simulink model "simulation_prev"  (R2021b)
settings: Solver=ode45  StartTime=0.0  StopTime=20.0  RelTol=1e-3
model workspace (MAT data in the model file):
  instants = 1
values from neighbouring files (symbols this model uses):
  c = modNE(x2,x2,e0,m,I,A,pc)    [ct_dynamics.m]    (also in dynamic_model_3R_spatial.m = [c1;c2;c3]; dynamic_model_simulation.m = [0.4; 0.2; 0.7]; run_experiment.m = [0.4; 0.2; 0.7])
  c0bar = norm(get_c_factorization_matrix(sol(1),sol(2),sol(3),sol(4),sol(5)))/norm(sol(3:5))    [compute_vel_obs_gain.m]    (also in dynamic_model_simulation.m = 1.96239028072; red_obs_gain_computation.m = c0; run_experiment.m = 1.96239028072)
  DHTABLE = [ pi/2      0         l(1)     q1 ... (first row only)    [compute_vel_obs_gain.m]    (also in dynamic_model_3R_spatial.m = [ pi/2      0      sym('L1') sym('q1'); dynamic_model_simulation.m = [ pi/2      0         l(1)     0; red_obs_gain_computation.m = [ pi/2      0         l(1)     0; run_experiment.m = [ pi/2      0         l(1)     0)
  eta = 1    [compute_vel_obs_gain.m]    (also in dynamic_model_simulation.m; red_obs_gain_computation.m; run_experiment.m)
  g0 = 9.81    [compute_vel_obs_gain.m]    (also in dynamic_model_3R_spatial.m; dynamic_model_simulation.m; modNE.m = 0; red_obs_gain_computation.m)
  I = zeros(3,3,N)    [compute_vel_obs_gain.m]    (also in dynamic_model_simulation.m; red_obs_gain_computation.m; run_experiment.m; run_simulation.m = zeros(3,3,3))
  K0 = c0bar*(v_max+eta)/(2*lambda_1)    [compute_vel_obs_gain.m]    (also in dynamic_model_simulation.m = 31.0539244645; red_obs_gain_computation.m = 0; run_experiment.m = 103.513081548)
  Kd = 3e1    (= 30)    [dynamic_model_simulation.m]    (also in run_experiment.m = 70; run_simulation.m = 10)
  Ko = 5e1    (= 50)    [dynamic_model_simulation.m]    (also in run_experiment.m; run_simulation.m = 0.1)
  Kp = 3e2    (= 300)    [dynamic_model_simulation.m]    (also in run_experiment.m = 70; run_simulation.m = 50)
  l = [0.5 0.5 0.4]'    [compute_eeJacobian.m]    (also in compute_vel_obs_gain.m; dynamic_model_simulation.m; eeJacobian_3R_spatial.m; red_obs_gain_computation.m)
  lambda_1 = min(min_first,min_third)/2    [compute_vel_obs_gain.m]    (also in dynamic_model_simulation.m = 0.0947894822263; red_obs_gain_computation.m = min_eig/2; run_experiment.m = 0.0473947411131)
  m = [15 10 5]'    [compute_vel_obs_gain.m]    (also in dynamic_model_simulation.m; red_obs_gain_computation.m; run_experiment.m; run_simulation.m = [m1 m2 m3]')
  pc = [0             -l(2)+dc(2) -l(3)+dc(3) ... (first row only)    [compute_vel_obs_gain.m]    (also in dynamic_model_simulation.m; red_obs_gain_computation.m; run_experiment.m)
  q0 = inverse_kinematics(p_init,l,soln_type)    [dynamic_model_simulation.m]    (also in run_experiment.m; run_simulation.m = [0,0,0]')
  r_c = 0.3    [dynamic_model_simulation.m]    (also in run_experiment.m)
  s0 = ceil(norm(dq0)/vbar)    [dynamic_model_simulation.m]
  T = simplify(T)    [DHMatrix.m]    (also in DHMatrix_sym.m; dynamic_model_3R_spatial.m = simplify(T1+T2+T3); dynamic_model_simulation.m = 2; run_experiment.m = 2)
  t0 = 2    [dynamic_model_simulation.m]    (also in run_experiment.m)
  T0 = 0.5*x2hat0'*M0*x2hat0    [dynamic_model_simulation.m]    (also in run_experiment.m)
  vbar = 2*eta+1    (= 3)    [dynamic_model_simulation.m]
  x0 = [pi/4,pi/4,1,1,1]'    [compute_vel_obs_gain.m]    (also in dynamic_model_simulation.m = [q0; dq0]; find_c0.m; run_experiment.m = [q0; dq0])
  z0 = [0 0 1]'    [dynamic_model_3R_spatial.m]    (also in dynamic_model_simulation.m = x2hat0 - K0*q0; run_experiment.m = x2hat0 - K0*q0)
undefined symbols (not defined in the file or in its folder): Levenberg, Marquardt, p_f, p_i, t_fin, t_init, time_int, trvec2tform
libraries: robotcorelib x3, SignalEditorBlockLib x1, robotmaniplib x1, matrix_library x1
(part 1 of 2)
settings Model: Creator=PcWork  LastModifiedBy=mluser
settings DataIOCC: SaveFormat=Array  SaveState=on
settings DebuggingCC: UnconnectedInputMsg=none  UnconnectedOutputMsg=none  UnconnectedLineMsg=none
settings RTWCC: DLArmComputeVersion=20.02.1

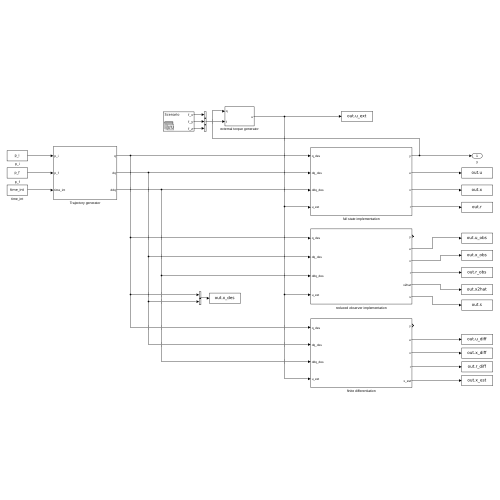
[thumbnail: Simulink's stored preview of the top-level diagram]
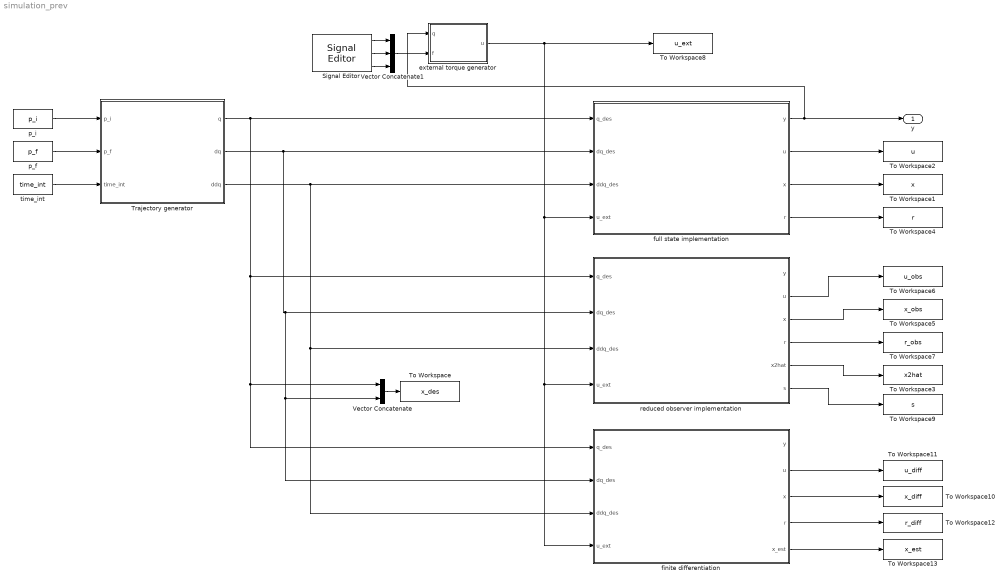
== system simulation_prev ==
  Signal Editor : SignalEditorBlockLib/Signal Editor  FileName=external_force.mat  ActiveScenario=Scenario  ActiveSignal=f_y  IsBus=off  OutputBusObjectStr=Bus: BusObject  SampleTime=0  ZeroCross=off  OutputAfterFinalValue=Setting to zero  Unit=inherit  PreserveSignalName=on
  To Workspace : ToWorkspace  VariableName=x_des  SampleTime=-1
  To Workspace1 : ToWorkspace  VariableName=x  SampleTime=-1
  To Workspace10 : ToWorkspace  VariableName=x_diff  SampleTime=-1
  To Workspace11 : ToWorkspace  VariableName=u_diff  SampleTime=-1
  To Workspace12 : ToWorkspace  VariableName=r_diff  SampleTime=-1
  To Workspace13 : ToWorkspace  VariableName=x_est  SampleTime=-1
  To Workspace2 : ToWorkspace  VariableName=u  SampleTime=-1
  To Workspace3 : ToWorkspace  VariableName=x2hat  SampleTime=-1
  To Workspace4 : ToWorkspace  VariableName=r  SampleTime=-1
  To Workspace5 : ToWorkspace  VariableName=x_obs  SampleTime=-1
  To Workspace6 : ToWorkspace  VariableName=u_obs  SampleTime=-1
  To Workspace7 : ToWorkspace  VariableName=r_obs  SampleTime=-1
  To Workspace8 : ToWorkspace  VariableName=u_ext  SampleTime=-1
  To Workspace9 : ToWorkspace  VariableName=s  SampleTime=-1
  Trajectory generator : Subsystem
  Vector Concatenate : Concatenate
  Vector Concatenate1 : Concatenate  NumInputs=3
  external torque generator : Subsystem
  finite differentiation : Subsystem
  full state implementation : Subsystem
  p_f : Constant  Value=p_f
  p_i : Constant  Value=p_i
  reduced observer implementation : Subsystem
  time_int : Constant  Value=time_int
  y : Outport
  wires:
  full state implementation/2(u) -> To Workspace2/1
  full state implementation/4(r) -> To Workspace4/1
  full state implementation/1(y) -> y/1, external torque generator/1(q)
  Vector Concatenate/1 -> To Workspace/1
  full state implementation/3(x) -> To Workspace1/1
  reduced observer implementation/2(u) -> To Workspace6/1
  reduced observer implementation/3(x) -> To Workspace5/1
  reduced observer implementation/4(r) -> To Workspace7/1
  external torque generator/1(u) -> finite differentiation/4(u_ext), reduced observer implementation/4(u_ext), full state implementation/4(u_ext), To Workspace8/1
  reduced observer implementation/5(x2hat) -> To Workspace3/1
  reduced observer implementation/6(s) -> To Workspace9/1
  finite differentiation/2(u) -> To Workspace11/1
  finite differentiation/3(x) -> To Workspace10/1
  finite differentiation/4(r) -> To Workspace12/1
  finite differentiation/5(x_est) -> To Workspace13/1
  Signal Editor/2 -> Vector Concatenate1/2
  Signal Editor/3 -> Vector Concatenate1/3
  Vector Concatenate1/1 -> external torque generator/2(f)
  Signal Editor/1 -> Vector Concatenate1/1
  p_i/1 -> Trajectory generator/1(p_i)
  p_f/1 -> Trajectory generator/2(p_f)
  time_int/1 -> Trajectory generator/3(time_int)
  Trajectory generator/1(q) -> finite differentiation/1(q_des), Vector Concatenate/1, reduced observer implementation/1(q_des), full state implementation/1(q_des)
  Trajectory generator/2(dq) -> full state implementation/2(dq_des), reduced observer implementation/2(dq_des), finite differentiation/2(dq_des), Vector Concatenate/2
  Trajectory generator/3(ddq) -> full state implementation/3(ddq_des), finite differentiation/3(ddq_des), reduced observer implementation/3(ddq_des)

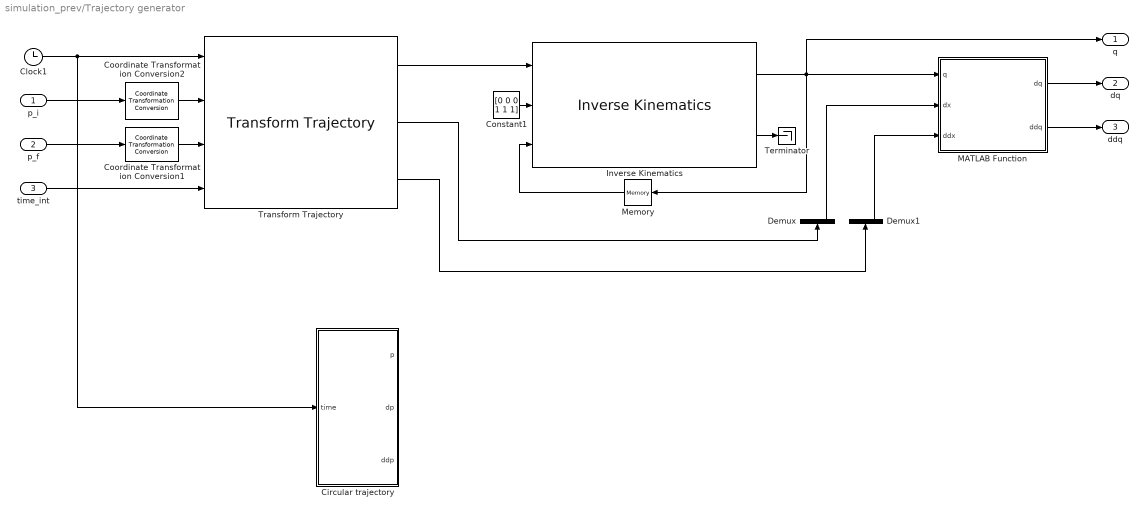
== system simulation_prev/Trajectory generator ==
  p_i : Inport
  p_f : Inport  Port=2
  time_int : Inport  Port=3
  Circular trajectory : Subsystem
  Clock1 : Clock
  Constant1 : Constant  Value=[0 0 0 1 1 1]
  Coordinate Transformation Conversion1 : robotcorelib/Coordinate Transformation Conversion  InputRepresentation=Translation Vector  InputEulerSequence=ZYX  ShowTrVecInputPort=on  OutputRepresentation=Homogeneous Transformation  OutputEulerSequence=ZYX  ShowTrVecOutputPort=on  SimulateUsing=Interpreted execution
  Coordinate Transformation Conversion2 : robotcorelib/Coordinate Transformation Conversion  InputRepresentation=Translation Vector  InputEulerSequence=ZYX  ShowTrVecInputPort=on  OutputRepresentation=Homogeneous Transformation  OutputEulerSequence=ZYX  ShowTrVecOutputPort=on  SimulateUsing=Interpreted execution
  Demux : Demux  Outputs=2
  Demux1 : Demux  Outputs=2
  Inverse Kinematics : robotmaniplib/Inverse Kinematics  RigidBodyTree=robot  EndEffector=body3  ShowInfo=on  SolverName=Levenberg-Marquardt  EnforceJointLimits=on  MaxIterations=1500  MaxTime=10  GradientTolerance=1e-3  SolutionTolerance=1e-2  StepTolerance=1e-14  ErrorChangeTolerance=1e-3  UseErrorDamping=on  DampingBias=0.0025  SimulateUsing=Interpreted execution
  MATLAB Function : MATLAB Function  TreatAsAtomicUnit=on
  Memory : Memory  InitialCondition=q0  InheritSampleTime=on
  Terminator : Terminator
  Transform Trajectory : robotcorelib/Transform Trajectory  WaypointSource=External  T0=trvec2tform(p_i)  TF=trvec2tform(p_f)  TimeInterval=time_int  CustomTimeScaling=off  ParameterSource=Internal  TSTime=2:0.1:3  TimeScaling=[ 0:0.1:1; ones( 1, 11 ); zeros( 1, 11 ) ]  SimulateUsing=Interpreted execution
  q : Outport
  dq : Outport  Port=2
  ddq : Outport  Port=3
  wires:
  time_int/1 -> Transform Trajectory/4
  Inverse Kinematics/1 -> q/1, MATLAB Function/1(q), Memory/1
  Transform Trajectory/1 -> Inverse Kinematics/1
  Demux/2 -> MATLAB Function/2(dx)
  Transform Trajectory/3 -> Demux1/1
  MATLAB Function/2(ddq) -> ddq/1
  MATLAB Function/1(dq) -> dq/1
  p_f/1 -> Coordinate Transformation Conversion1/1
  Clock1/1 -> Circular trajectory/1(time), Transform Trajectory/1
  p_i/1 -> Coordinate Transformation Conversion2/1
  Coordinate Transformation Conversion2/1 -> Transform Trajectory/2
  Coordinate Transformation Conversion1/1 -> Transform Trajectory/3
  Memory/1 -> Inverse Kinematics/3
  Transform Trajectory/2 -> Demux/1
  Demux1/2 -> MATLAB Function/3(ddx)
  Constant1/1 -> Inverse Kinematics/2
  Inverse Kinematics/2 -> Terminator/1

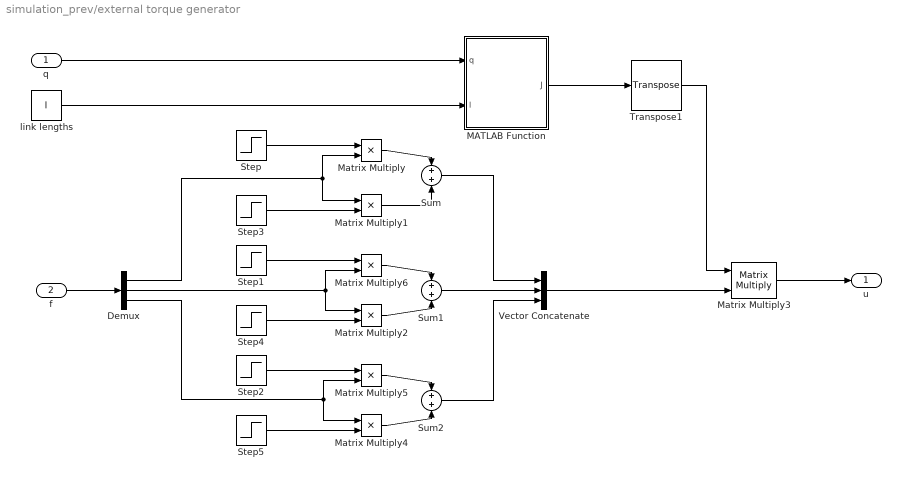
== system simulation_prev/external torque generator ==
  q : Inport
  f : Inport  Port=2
  Demux : Demux  Outputs=3
  MATLAB Function : MATLAB Function  TreatAsAtomicUnit=on
  Matrix Multiply{,1..2,4..6} (6 alike) : Product
  Matrix Multiply3 : Product  Multiplication=Matrix(*)
  Step : Step  Time=t_init  SampleTime=0
  Step1 : Step  Time=t_init  SampleTime=0
  Step2 : Step  Time=t_init  SampleTime=0
  Step3 : Step  Time=t_fin  After=-1  SampleTime=0
  Step4 : Step  Time=t_fin  After=-1  SampleTime=0
  Step5 : Step  Time=t_fin  After=-1  SampleTime=0
  Sum : Sum
  Sum1 : Sum
  Sum2 : Sum
  Transpose1 : matrix_library/Transpose
  Vector Concatenate : Concatenate  NumInputs=3
  link lengths : Constant  Value=l
  u : Outport
  wires:
  Step1/1 -> Matrix Multiply6/1
  Demux/2 -> Matrix Multiply2/1, Matrix Multiply6/2
  Demux/1 -> Matrix Multiply1/1, Matrix Multiply/2
  f/1 -> Demux/1
  MATLAB Function/1(J) -> Transpose1/1
  Transpose1/1 -> Matrix Multiply3/1
  Vector Concatenate/1 -> Matrix Multiply3/2
  Matrix Multiply3/1 -> u/1
  q/1 -> MATLAB Function/1(q)
  link lengths/1 -> MATLAB Function/2(l)
  Step3/1 -> Matrix Multiply1/2
  Step4/1 -> Matrix Multiply2/2
  Step/1 -> Matrix Multiply/1
  Matrix Multiply1/1 -> Sum/2
  Sum/1 -> Vector Concatenate/1
  Matrix Multiply/1 -> Sum/1
  Matrix Multiply6/1 -> Sum1/1
  Matrix Multiply2/1 -> Sum1/2
  Sum1/1 -> Vector Concatenate/2
  Step5/1 -> Matrix Multiply4/2
  Matrix Multiply5/1 -> Sum2/1
  Demux/3 -> Matrix Multiply5/2, Matrix Multiply4/1
  Matrix Multiply4/1 -> Sum2/2
  Step2/1 -> Matrix Multiply5/1
  Sum2/1 -> Vector Concatenate/3

== system simulation_prev/finite differentiation ==
  q_des : Inport
  dq_des : Inport  Port=2
  ddq_des : Inport  Port=3
  u_ext : Inport  Port=4
  Controller : Subsystem
  Demux1 : Demux  Outputs=2
  Derivative : Derivative
  Robot dynamics : Subsystem
  Sum : Sum
  Terminator : Terminator
  Vector Concatenate : Concatenate
  energy residual : Subsystem
  y : Outport
  u : Outport  Port=2
  x : Outport  Port=3
  r : Outport  Port=4
  x_est : Outport  Port=5
  wires:
  Demux1/1 -> Derivative/1, Vector Concatenate/1, y/1
  energy residual/1(r) -> r/1
  q_des/1 -> Controller/2(q_des)
  Controller/1(u) -> energy residual/2(u_m), Sum/1, u/1
  ddq_des/1 -> Controller/4(ddq_des)
  Demux1/2 -> Terminator/1
  dq_des/1 -> Controller/3(dq_des)
  Robot dynamics/1(x) -> x/1, Demux1/1
  Vector Concatenate/1 -> x_est/1, energy residual/1(x), Controller/1(x)
  Sum/1 -> Robot dynamics/1(u)
  u_ext/1 -> Sum/2
  Derivative/1 -> Vector Concatenate/2

== system simulation_prev/full state implementation ==
  q_des : Inport
  dq_des : Inport  Port=2
  ddq_des : Inport  Port=3
  u_ext : Inport  Port=4
  Controller : Subsystem
  Demux1 : Demux  Outputs=2
  Robot dynamics : Subsystem
  Sum : Sum
  Terminator : Terminator
  energy residual : Subsystem
  y : Outport
  u : Outport  Port=2
  x : Outport  Port=3
  r : Outport  Port=4
  wires:
  Demux1/2 -> Terminator/1
  Robot dynamics/1(x) -> energy residual/1(x), x/1, Demux1/1, Controller/1(x)
  energy residual/1(r) -> r/1
  Sum/1 -> Robot dynamics/1(u)
  q_des/1 -> Controller/2(q_des)
  Controller/1(u) -> u/1, Sum/1, energy residual/2(u_m)
  dq_des/1 -> Controller/3(dq_des)
  ddq_des/1 -> Controller/4(ddq_des)
  Demux1/1 -> y/1
  u_ext/1 -> Sum/2

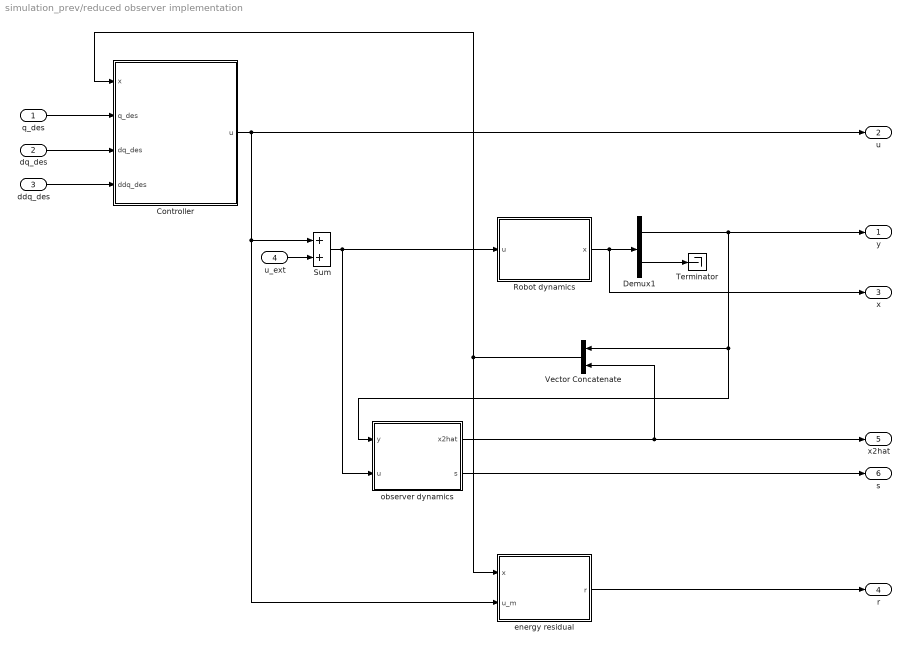
== system simulation_prev/reduced observer implementation ==
  q_des : Inport
  dq_des : Inport  Port=2
  ddq_des : Inport  Port=3
  u_ext : Inport  Port=4
  Controller : Subsystem
  Demux1 : Demux  Outputs=2
  Robot dynamics : Subsystem
  Sum : Sum
  Terminator : Terminator
  Vector Concatenate : Concatenate
  energy residual : Subsystem
  observer dynamics : Subsystem
  y : Outport
  u : Outport  Port=2
  x : Outport  Port=3
  r : Outport  Port=4
  x2hat : Outport  Port=5
  s : Outport  Port=6
  wires:
  Demux1/1 -> Vector Concatenate/1, observer dynamics/1(y), y/1
  observer dynamics/1(x2hat) -> x2hat/1, Vector Concatenate/2
  energy residual/1(r) -> r/1
  q_des/1 -> Controller/2(q_des)
  Controller/1(u) -> energy residual/2(u_m), Sum/1, u/1
  ddq_des/1 -> Controller/4(ddq_des)
  Demux1/2 -> Terminator/1
  dq_des/1 -> Controller/3(dq_des)
  Robot dynamics/1(x) -> x/1, Demux1/1
  Vector Concatenate/1 -> energy residual/1(x), Controller/1(x)
  Sum/1 -> Robot dynamics/1(u), observer dynamics/2(u)
  u_ext/1 -> Sum/2
  observer dynamics/2(s) -> s/1

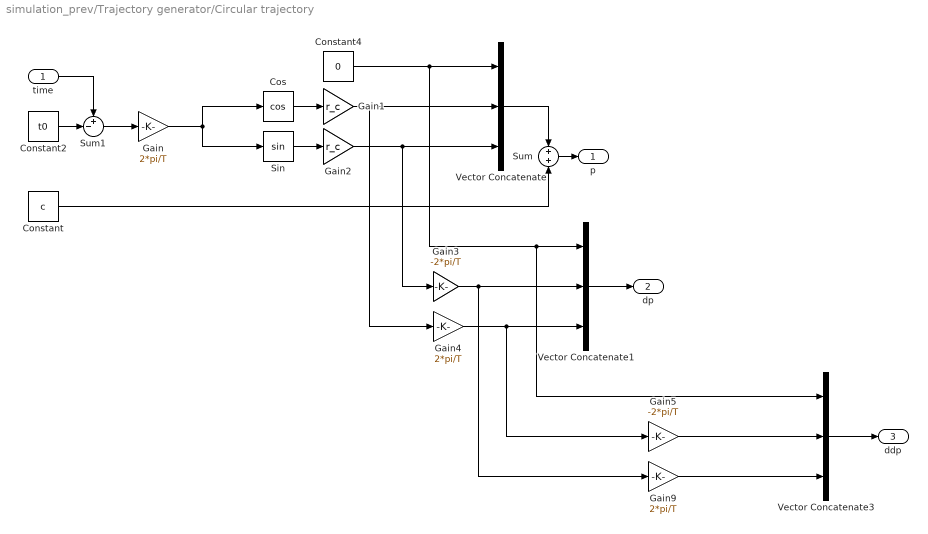
== system simulation_prev/Trajectory generator/Circular trajectory ==
  time : Inport
  Constant : Constant  Value=c
  Constant2 : Constant  Value=t0
  Constant4 : Constant  Value=0
  Cos : Trigonometry  Operator=cos
  Gain : Gain  Gain=2*pi/T
  Gain1 : Gain  Gain=r_c
  Gain2 : Gain  Gain=r_c
  Gain3 : Gain  Gain=-2*pi/T
  Gain4 : Gain  Gain=2*pi/T
  Gain5 : Gain  Gain=-2*pi/T
  Gain9 : Gain  Gain=2*pi/T
  Sin : Trigonometry
  Sum : Sum
  Sum1 : Sum  Inputs=+-|
  Vector Concatenate : Concatenate  NumInputs=3
  Vector Concatenate1 : Concatenate  NumInputs=3
  Vector Concatenate3 : Concatenate  NumInputs=3
  p : Outport
  dp : Outport  Port=2
  ddp : Outport  Port=3
  wires:
  Constant2/1 -> Sum1/2
  Sum/1 -> p/1
  Sum1/1 -> Gain/1
  Constant4/1 -> Vector Concatenate3/1, Vector Concatenate1/1, Vector Concatenate/1
  Gain2/1 -> Vector Concatenate/3, Gain3/1
  Constant/1 -> Sum/2
  time/1 -> Sum1/1
  Cos/1 -> Gain1/1
  Gain/1 -> Sin/1, Cos/1
  Sin/1 -> Gain2/1
  Vector Concatenate/1 -> Sum/1
  Gain1/1 -> Vector Concatenate/2, Gain4/1
  Gain3/1 -> Gain9/1, Vector Concatenate1/2
  Gain4/1 -> Gain5/1, Vector Concatenate1/3
  Gain9/1 -> Vector Concatenate3/3
  Gain5/1 -> Vector Concatenate3/2
  Vector Concatenate3/1 -> ddp/1
  Vector Concatenate1/1 -> dp/1

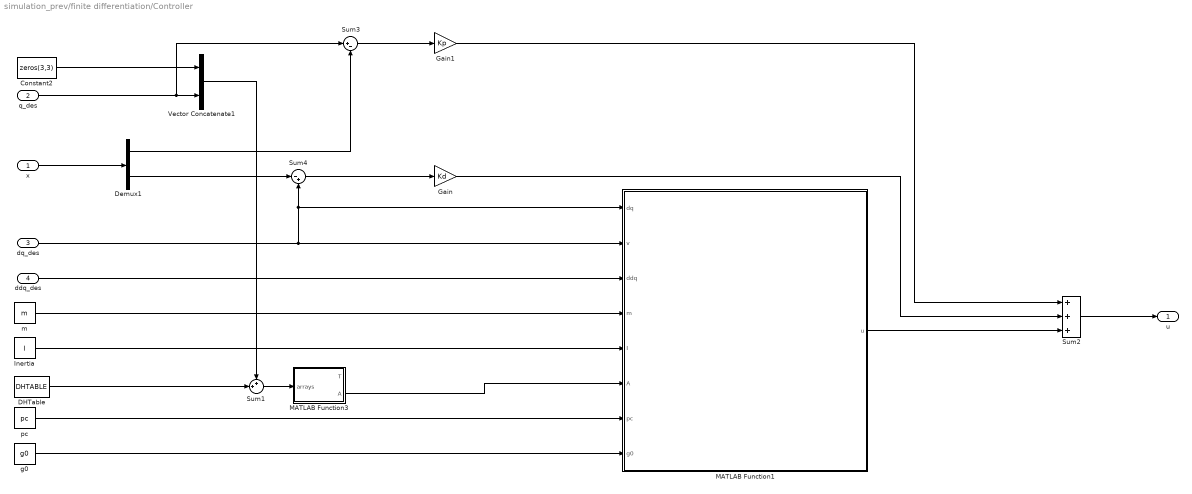
== system simulation_prev/finite differentiation/Controller ==
  x : Inport
  q_des : Inport  Port=2
  dq_des : Inport  Port=3
  ddq_des : Inport  Port=4
  Constant2 : Constant  Value=zeros(3,3)
  DHTable : Constant  Value=DHTABLE
  Demux1 : Demux  Outputs=2
  Gain : Gain  Gain=Kd
  Gain1 : Gain  Gain=Kp
  Inertia : Constant  Value=I
  MATLAB Function1 : MATLAB Function  TreatAsAtomicUnit=on
  MATLAB Function3 : MATLAB Function  TreatAsAtomicUnit=on
  Sum1 : Sum  Inputs=++|
  Sum2 : Sum  Inputs=+++
  Sum3 : Sum  Inputs=|+-
  Sum4 : Sum  Inputs=|-+
  Vector Concatenate1 : Concatenate  Mode=Multidimensional array  ConcatenateDimension=2
  g0 : Constant  Value=g0
  m : Constant  Value=m
  pc : Constant  Value=pc
  u : Outport
  wires:
  MATLAB Function3/2(A) -> MATLAB Function1/6(A)
  dq_des/1 -> MATLAB Function1/1(dq), Sum4/2, MATLAB Function1/2(v)
  ddq_des/1 -> MATLAB Function1/3(ddq)
  Sum1/1 -> MATLAB Function3/1(arrays)
  Constant2/1 -> Vector Concatenate1/1
  Sum4/1 -> Gain/1
  Vector Concatenate1/1 -> Sum1/1
  m/1 -> MATLAB Function1/4(m)
  g0/1 -> MATLAB Function1/8(g0)
  Sum3/1 -> Gain1/1
  q_des/1 -> Vector Concatenate1/2, Sum3/1
  DHTable/1 -> Sum1/2
  Inertia/1 -> MATLAB Function1/5(I)
  pc/1 -> MATLAB Function1/7(pc)
  Sum2/1 -> u/1
  MATLAB Function1/1(u) -> Sum2/3
  Gain/1 -> Sum2/2
  Gain1/1 -> Sum2/1
  x/1 -> Demux1/1
  Demux1/2 -> Sum4/1
  Demux1/1 -> Sum3/2

== system simulation_prev/finite differentiation/Robot dynamics ==
  u : Inport
  Constant : Constant  Value=zeros(3,3)
  DHTable : Constant  Value=DHTABLE
  Demux1 : Demux  Outputs=2
  Inertia : Constant  Value=I
  Integrator : Integrator  InitialConditionSource=external  InitialCondition=[0 pi/4 pi/4 0 0 0]'
  MATLAB Function : MATLAB Function  TreatAsAtomicUnit=on
  MATLAB Function2 : MATLAB Function  TreatAsAtomicUnit=on
  Sum : Sum
  Vector Concatenate : Concatenate  Mode=Multidimensional array  ConcatenateDimension=2
  g0 : Constant  Value=g0
  m : Constant  Value=m
  pc : Constant  Value=pc
  x0 : Constant  Value=x0
  x : Outport
  wires:
  Vector Concatenate/1 -> Sum/1
  Constant/1 -> Vector Concatenate/1
  Integrator/1 -> Demux1/1, MATLAB Function/1(x), x/1
  MATLAB Function/1(dx) -> Integrator/1
  x0/1 -> Integrator/2
  u/1 -> MATLAB Function/2(u)
  Sum/1 -> MATLAB Function2/1(arrays)
  MATLAB Function2/2(A) -> MATLAB Function/5(A)
  DHTable/1 -> Sum/2
  pc/1 -> MATLAB Function/6(pc)
  m/1 -> MATLAB Function/3(m)
  Inertia/1 -> MATLAB Function/4(I)
  g0/1 -> MATLAB Function/7(g0)
  Demux1/1 -> Vector Concatenate/2

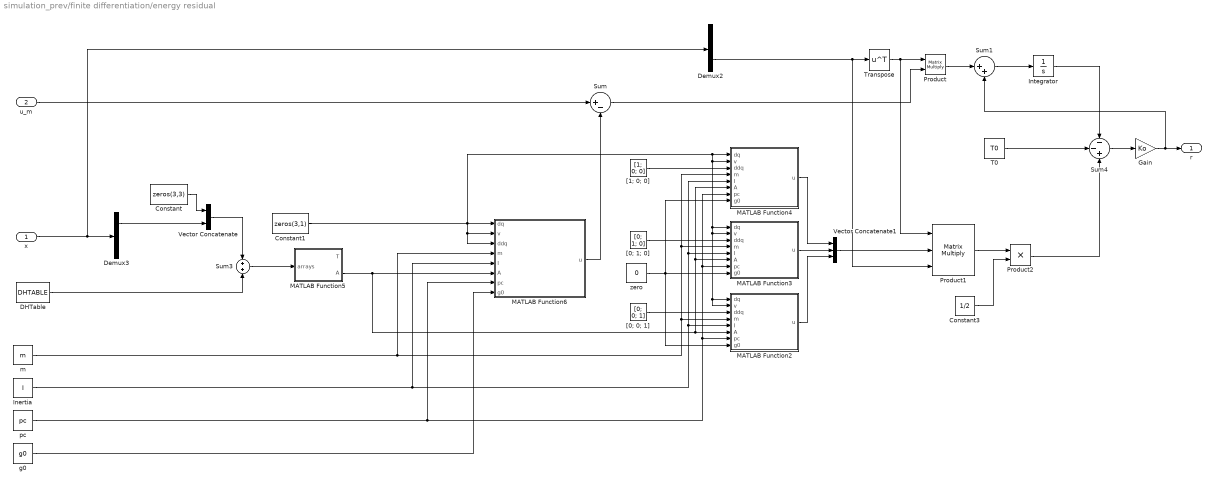
== system simulation_prev/finite differentiation/energy residual ==
  x : Inport
  u_m : Inport  Port=2
  Constant : Constant  Value=zeros(3,3)
  Constant1 : Constant  Value=zeros(3,1)
  Constant3 : Constant  Value=1/2
  DHTable : Constant  Value=DHTABLE
  Demux2 : Demux  Outputs=2
  Demux3 : Demux  Outputs=2
  Gain : Gain  Gain=Ko
  Inertia : Constant  Value=I
  Integrator : Integrator
  MATLAB Function2 : MATLAB Function  TreatAsAtomicUnit=on
  MATLAB Function3 : MATLAB Function  TreatAsAtomicUnit=on
  MATLAB Function4 : MATLAB Function  TreatAsAtomicUnit=on
  MATLAB Function5 : MATLAB Function  TreatAsAtomicUnit=on
  MATLAB Function6 : MATLAB Function  TreatAsAtomicUnit=on
  Product : Product  Multiplication=Matrix(*)
  Product1 : Product  Inputs=3  Multiplication=Matrix(*)
  Product2 : Product
  Sum : Sum  Inputs=|+-
  Sum1 : Sum  Inputs=|++
  Sum3 : Sum
  Sum4 : Sum  Inputs=--+
  T0 : Constant  Value=T0
  Transpose : Math  Operator=transpose  SaturateOnIntegerOverflow=on
  Vector Concatenate : Concatenate  Mode=Multidimensional array  ConcatenateDimension=2
  Vector Concatenate1 : Concatenate  NumInputs=3  Mode=Multidimensional array  ConcatenateDimension=2
  "[0; 0; 1]" : Constant  Value=[0; 0; 1]
  "[0; 1; 0]" : Constant  Value=[0; 1; 0]
  "[1; 0; 0]" : Constant  Value=[1; 0; 0]
  g0 : Constant  Value=g0
  m : Constant  Value=m
  pc : Constant  Value=pc
  zero : Constant  Value=0
  r : Outport
  wires:
  MATLAB Function2/1(u) -> Vector Concatenate1/3
  zero/1 -> MATLAB Function4/8(g0), MATLAB Function2/8(g0), MATLAB Function3/8(g0)
  MATLAB Function5/2(A) -> MATLAB Function6/6(A), MATLAB Function4/6(A), MATLAB Function3/6(A), MATLAB Function2/6(A)
  Sum/1 -> Product/2
  Sum1/1 -> Integrator/1
  T0/1 -> Sum4/2
  Vector Concatenate/1 -> Sum3/1
  Inertia/1 -> MATLAB Function6/5(I), MATLAB Function4/5(I), MATLAB Function3/5(I), MATLAB Function2/5(I)
  Sum4/1 -> Gain/1
  Constant/1 -> Vector Concatenate/1
  Gain/1 -> Sum1/2, r/1
  Sum3/1 -> MATLAB Function5/1(arrays)
  Constant1/1 -> MATLAB Function6/1(dq), MATLAB Function2/2(v), MATLAB Function2/1(dq), MATLAB Function3/2(v), MATLAB Function3/1(dq), MATLAB Function4/2(v), MATLAB Function4/1(dq), MATLAB Function6/2(v), MATLAB Function6/3(ddq)
  Demux3/1 -> Vector Concatenate/2
  "[1; 0; 0]"/1 -> MATLAB Function4/3(ddq)
  MATLAB Function6/1(u) -> Sum/2
  x/1 -> Demux2/1, Demux3/1
  "[0; 1; 0]"/1 -> MATLAB Function3/3(ddq)
  u_m/1 -> Sum/1
  m/1 -> MATLAB Function2/4(m), MATLAB Function3/4(m), MATLAB Function4/4(m), MATLAB Function6/4(m)
  "[0; 0; 1]"/1 -> MATLAB Function2/3(ddq)
  Constant3/1 -> Product2/2
  MATLAB Function4/1(u) -> Vector Concatenate1/1
  DHTable/1 -> Sum3/2
  MATLAB Function3/1(u) -> Vector Concatenate1/2
  Product1/1 -> Product2/1
  Vector Concatenate1/1 -> Product1/2
  Product2/1 -> Sum4/3
  g0/1 -> MATLAB Function6/8(g0)
  Demux2/2 -> Product1/3, Transpose/1
  Transpose/1 -> Product1/1, Product/1
  pc/1 -> MATLAB Function6/7(pc), MATLAB Function4/7(pc), MATLAB Function3/7(pc), MATLAB Function2/7(pc)
  Product/1 -> Sum1/1
  Integrator/1 -> Sum4/1

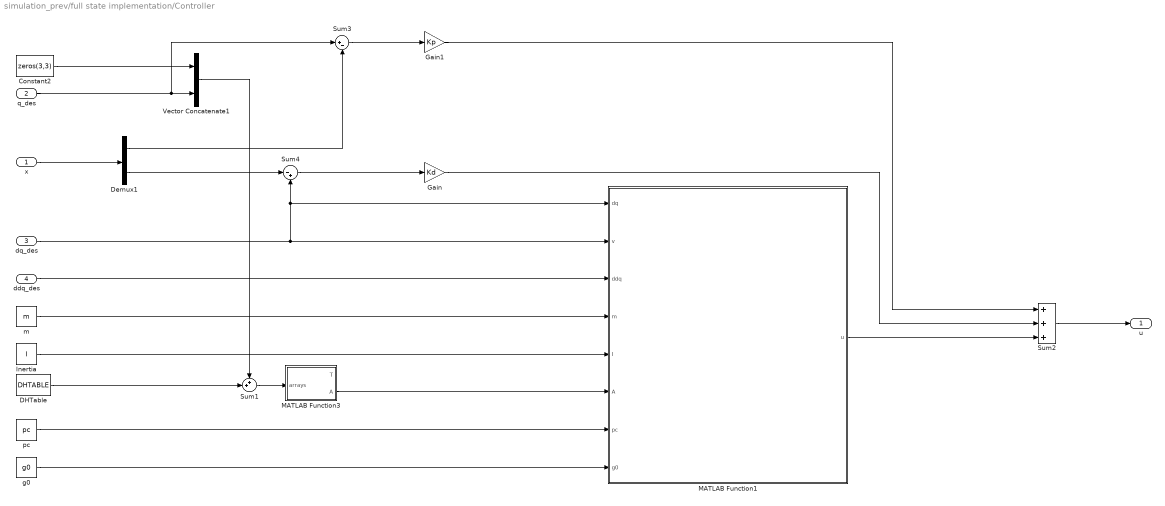
== system simulation_prev/full state implementation/Controller ==
  x : Inport
  q_des : Inport  Port=2
  dq_des : Inport  Port=3
  ddq_des : Inport  Port=4
  Constant2 : Constant  Value=zeros(3,3)
  DHTable : Constant  Value=DHTABLE
  Demux1 : Demux  Outputs=2
  Gain : Gain  Gain=Kd
  Gain1 : Gain  Gain=Kp
  Inertia : Constant  Value=I
  MATLAB Function1 : MATLAB Function  TreatAsAtomicUnit=on
  MATLAB Function3 : MATLAB Function  TreatAsAtomicUnit=on
  Sum1 : Sum  Inputs=++|
  Sum2 : Sum  Inputs=+++
  Sum3 : Sum  Inputs=|+-
  Sum4 : Sum  Inputs=|-+
  Vector Concatenate1 : Concatenate  Mode=Multidimensional array  ConcatenateDimension=2
  g0 : Constant  Value=g0
  m : Constant  Value=m
  pc : Constant  Value=pc
  u : Outport
  wires:
  MATLAB Function3/2(A) -> MATLAB Function1/6(A)
  dq_des/1 -> MATLAB Function1/1(dq), Sum4/2, MATLAB Function1/2(v)
  ddq_des/1 -> MATLAB Function1/3(ddq)
  Sum1/1 -> MATLAB Function3/1(arrays)
  Constant2/1 -> Vector Concatenate1/1
  Sum4/1 -> Gain/1
  Vector Concatenate1/1 -> Sum1/1
  m/1 -> MATLAB Function1/4(m)
  g0/1 -> MATLAB Function1/8(g0)
  Sum3/1 -> Gain1/1
  q_des/1 -> Vector Concatenate1/2, Sum3/1
  DHTable/1 -> Sum1/2
  Inertia/1 -> MATLAB Function1/5(I)
  pc/1 -> MATLAB Function1/7(pc)
  Sum2/1 -> u/1
  MATLAB Function1/1(u) -> Sum2/3
  Gain/1 -> Sum2/2
  Gain1/1 -> Sum2/1
  x/1 -> Demux1/1
  Demux1/2 -> Sum4/1
  Demux1/1 -> Sum3/2

== system simulation_prev/full state implementation/Robot dynamics ==
  u : Inport
  Constant : Constant  Value=zeros(3,3)
  DHTable : Constant  Value=DHTABLE
  Demux1 : Demux  Outputs=2
  Inertia : Constant  Value=I
  Integrator : Integrator  InitialConditionSource=external  InitialCondition=[0 pi/4 pi/4 0 0 0]'
  MATLAB Function : MATLAB Function  TreatAsAtomicUnit=on
  MATLAB Function2 : MATLAB Function  TreatAsAtomicUnit=on
  Sum : Sum
  Vector Concatenate : Concatenate  Mode=Multidimensional array  ConcatenateDimension=2
  g0 : Constant  Value=g0
  m : Constant  Value=m
  pc : Constant  Value=pc
  x0 : Constant  Value=x0
  x : Outport
  wires:
  Vector Concatenate/1 -> Sum/1
  Constant/1 -> Vector Concatenate/1
  Integrator/1 -> x/1, Demux1/1, MATLAB Function/1(x)
  MATLAB Function/1(dx) -> Integrator/1
  x0/1 -> Integrator/2
  u/1 -> MATLAB Function/2(u)
  Sum/1 -> MATLAB Function2/1(arrays)
  MATLAB Function2/2(A) -> MATLAB Function/5(A)
  DHTable/1 -> Sum/2
  pc/1 -> MATLAB Function/6(pc)
  m/1 -> MATLAB Function/3(m)
  Inertia/1 -> MATLAB Function/4(I)
  g0/1 -> MATLAB Function/7(g0)
  Demux1/1 -> Vector Concatenate/2

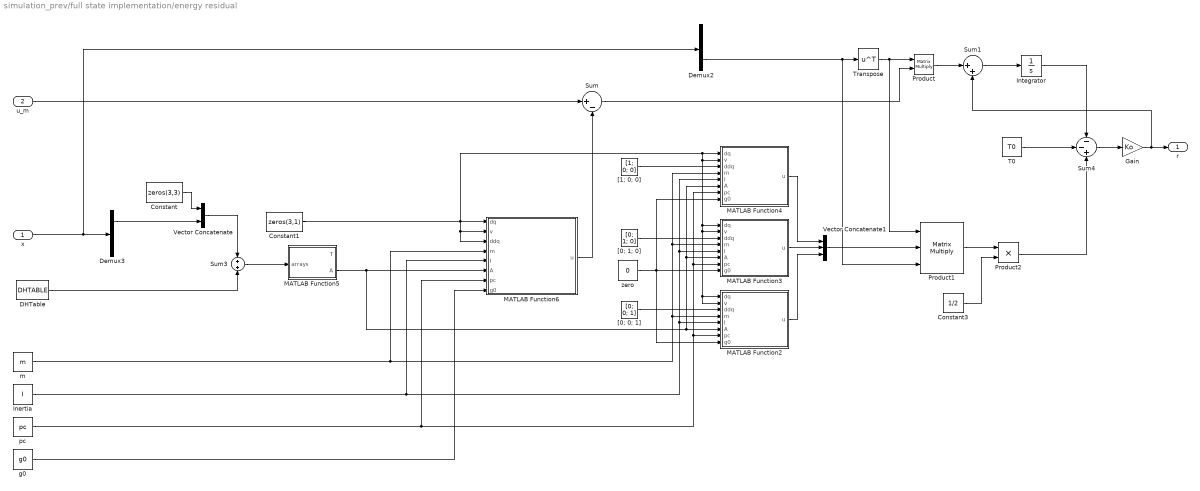
== system simulation_prev/full state implementation/energy residual ==
  x : Inport
  u_m : Inport  Port=2
  Constant : Constant  Value=zeros(3,3)
  Constant1 : Constant  Value=zeros(3,1)
  Constant3 : Constant  Value=1/2
  DHTable : Constant  Value=DHTABLE
  Demux2 : Demux  Outputs=2
  Demux3 : Demux  Outputs=2
  Gain : Gain  Gain=Ko
  Inertia : Constant  Value=I
  Integrator : Integrator
  MATLAB Function2 : MATLAB Function  TreatAsAtomicUnit=on
  MATLAB Function3 : MATLAB Function  TreatAsAtomicUnit=on
  MATLAB Function4 : MATLAB Function  TreatAsAtomicUnit=on
  MATLAB Function5 : MATLAB Function  TreatAsAtomicUnit=on
  MATLAB Function6 : MATLAB Function  TreatAsAtomicUnit=on
  Product : Product  Multiplication=Matrix(*)
  Product1 : Product  Inputs=3  Multiplication=Matrix(*)
  Product2 : Product
  Sum : Sum  Inputs=|+-
  Sum1 : Sum  Inputs=|++
  Sum3 : Sum
  Sum4 : Sum  Inputs=--+
  T0 : Constant  Value=T0
  Transpose : Math  Operator=transpose  SaturateOnIntegerOverflow=on
  Vector Concatenate : Concatenate  Mode=Multidimensional array  ConcatenateDimension=2
  Vector Concatenate1 : Concatenate  NumInputs=3  Mode=Multidimensional array  ConcatenateDimension=2
  "[0; 0; 1]" : Constant  Value=[0; 0; 1]
  "[0; 1; 0]" : Constant  Value=[0; 1; 0]
  "[1; 0; 0]" : Constant  Value=[1; 0; 0]
  g0 : Constant  Value=g0
  m : Constant  Value=m
  pc : Constant  Value=pc
  zero : Constant  Value=0
  r : Outport
  wires:
  MATLAB Function2/1(u) -> Vector Concatenate1/3
  zero/1 -> MATLAB Function4/8(g0), MATLAB Function2/8(g0), MATLAB Function3/8(g0)
  MATLAB Function5/2(A) -> MATLAB Function6/6(A), MATLAB Function4/6(A), MATLAB Function3/6(A), MATLAB Function2/6(A)
  Sum/1 -> Product/2
  Sum1/1 -> Integrator/1
  T0/1 -> Sum4/2
  Vector Concatenate/1 -> Sum3/1
  Inertia/1 -> MATLAB Function6/5(I), MATLAB Function4/5(I), MATLAB Function3/5(I), MATLAB Function2/5(I)
  Sum4/1 -> Gain/1
  Constant/1 -> Vector Concatenate/1
  Gain/1 -> Sum1/2, r/1
  Sum3/1 -> MATLAB Function5/1(arrays)
  Constant1/1 -> MATLAB Function6/1(dq), MATLAB Function2/2(v), MATLAB Function2/1(dq), MATLAB Function3/2(v), MATLAB Function3/1(dq), MATLAB Function4/2(v), MATLAB Function4/1(dq), MATLAB Function6/2(v), MATLAB Function6/3(ddq)
  Demux3/1 -> Vector Concatenate/2
  "[1; 0; 0]"/1 -> MATLAB Function4/3(ddq)
  MATLAB Function6/1(u) -> Sum/2
  x/1 -> Demux2/1, Demux3/1
  "[0; 1; 0]"/1 -> MATLAB Function3/3(ddq)
  u_m/1 -> Sum/1
  m/1 -> MATLAB Function6/4(m), MATLAB Function2/4(m), MATLAB Function3/4(m), MATLAB Function4/4(m)
  "[0; 0; 1]"/1 -> MATLAB Function2/3(ddq)
  Constant3/1 -> Product2/2
  MATLAB Function4/1(u) -> Vector Concatenate1/1
  DHTable/1 -> Sum3/2
  MATLAB Function3/1(u) -> Vector Concatenate1/2
  Product1/1 -> Product2/1
  Vector Concatenate1/1 -> Product1/2
  Product2/1 -> Sum4/3
  g0/1 -> MATLAB Function6/8(g0)
  Demux2/2 -> Product1/3, Transpose/1
  Transpose/1 -> Product1/1, Product/1
  pc/1 -> MATLAB Function6/7(pc), MATLAB Function4/7(pc), MATLAB Function3/7(pc), MATLAB Function2/7(pc)
  Product/1 -> Sum1/1
  Integrator/1 -> Sum4/1

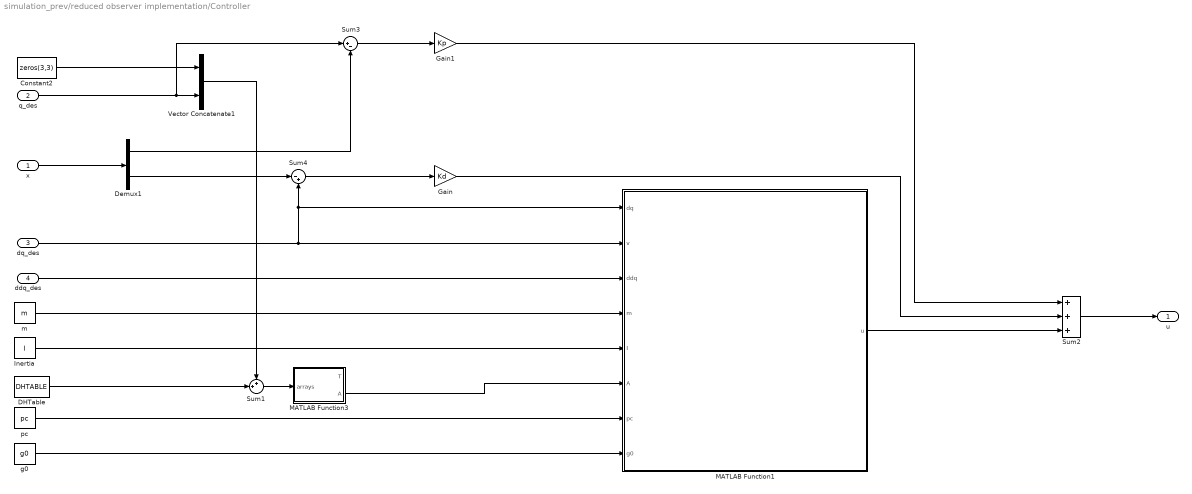
== system simulation_prev/reduced observer implementation/Controller ==
  x : Inport
  q_des : Inport  Port=2
  dq_des : Inport  Port=3
  ddq_des : Inport  Port=4
  Constant2 : Constant  Value=zeros(3,3)
  DHTable : Constant  Value=DHTABLE
  Demux1 : Demux  Outputs=2
  Gain : Gain  Gain=Kd
  Gain1 : Gain  Gain=Kp
  Inertia : Constant  Value=I
  MATLAB Function1 : MATLAB Function  TreatAsAtomicUnit=on
  MATLAB Function3 : MATLAB Function  TreatAsAtomicUnit=on
  Sum1 : Sum  Inputs=++|
  Sum2 : Sum  Inputs=+++
  Sum3 : Sum  Inputs=|+-
  Sum4 : Sum  Inputs=|-+
  Vector Concatenate1 : Concatenate  Mode=Multidimensional array  ConcatenateDimension=2
  g0 : Constant  Value=g0
  m : Constant  Value=m
  pc : Constant  Value=pc
  u : Outport
  wires:
  MATLAB Function3/2(A) -> MATLAB Function1/6(A)
  dq_des/1 -> MATLAB Function1/1(dq), Sum4/2, MATLAB Function1/2(v)
  ddq_des/1 -> MATLAB Function1/3(ddq)
  Sum1/1 -> MATLAB Function3/1(arrays)
  Constant2/1 -> Vector Concatenate1/1
  Sum4/1 -> Gain/1
  Vector Concatenate1/1 -> Sum1/1
  m/1 -> MATLAB Function1/4(m)
  g0/1 -> MATLAB Function1/8(g0)
  Sum3/1 -> Gain1/1
  q_des/1 -> Vector Concatenate1/2, Sum3/1
  DHTable/1 -> Sum1/2
  Inertia/1 -> MATLAB Function1/5(I)
  pc/1 -> MATLAB Function1/7(pc)
  Sum2/1 -> u/1
  MATLAB Function1/1(u) -> Sum2/3
  Gain/1 -> Sum2/2
  Gain1/1 -> Sum2/1
  x/1 -> Demux1/1
  Demux1/2 -> Sum4/1
  Demux1/1 -> Sum3/2

== system simulation_prev/reduced observer implementation/Robot dynamics ==
  u : Inport
  Constant : Constant  Value=zeros(3,3)
  DHTable : Constant  Value=DHTABLE
  Demux1 : Demux  Outputs=2
  Inertia : Constant  Value=I
  Integrator : Integrator  InitialConditionSource=external  InitialCondition=[0 pi/4 pi/4 0 0 0]'
  MATLAB Function : MATLAB Function  TreatAsAtomicUnit=on
  MATLAB Function2 : MATLAB Function  TreatAsAtomicUnit=on
  Sum : Sum
  Vector Concatenate : Concatenate  Mode=Multidimensional array  ConcatenateDimension=2
  g0 : Constant  Value=g0
  m : Constant  Value=m
  pc : Constant  Value=pc
  x0 : Constant  Value=x0
  x : Outport
  wires:
  Vector Concatenate/1 -> Sum/1
  Constant/1 -> Vector Concatenate/1
  Integrator/1 -> Demux1/1, MATLAB Function/1(x), x/1
  MATLAB Function/1(dx) -> Integrator/1
  x0/1 -> Integrator/2
  u/1 -> MATLAB Function/2(u)
  Sum/1 -> MATLAB Function2/1(arrays)
  MATLAB Function2/2(A) -> MATLAB Function/5(A)
  DHTable/1 -> Sum/2
  pc/1 -> MATLAB Function/6(pc)
  m/1 -> MATLAB Function/3(m)
  Inertia/1 -> MATLAB Function/4(I)
  g0/1 -> MATLAB Function/7(g0)
  Demux1/1 -> Vector Concatenate/2

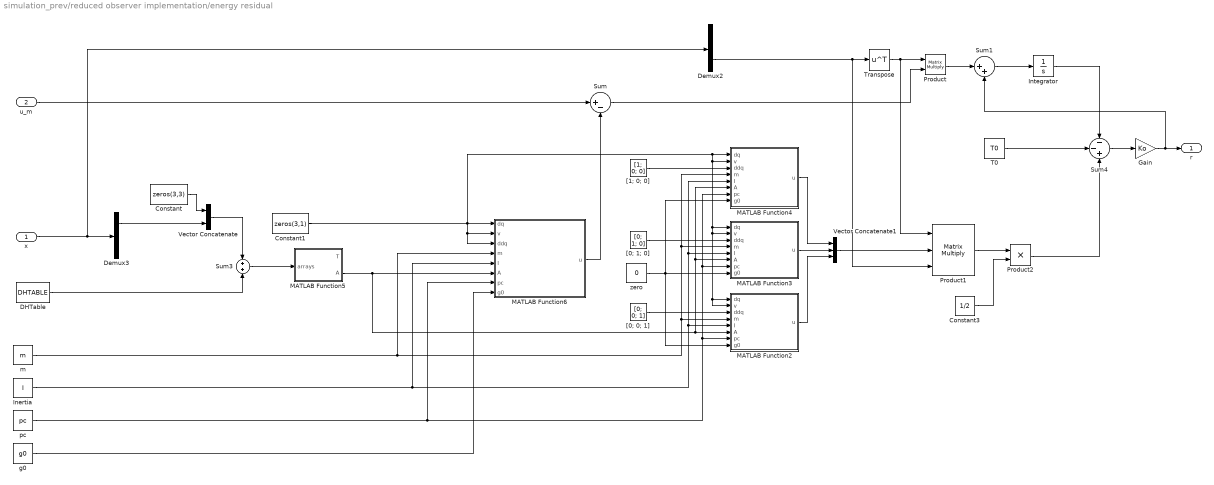
== system simulation_prev/reduced observer implementation/energy residual ==
  x : Inport
  u_m : Inport  Port=2
  Constant : Constant  Value=zeros(3,3)
  Constant1 : Constant  Value=zeros(3,1)
  Constant3 : Constant  Value=1/2
  DHTable : Constant  Value=DHTABLE
  Demux2 : Demux  Outputs=2
  Demux3 : Demux  Outputs=2
  Gain : Gain  Gain=Ko
  Inertia : Constant  Value=I
  Integrator : Integrator
  MATLAB Function2 : MATLAB Function  TreatAsAtomicUnit=on
  MATLAB Function3 : MATLAB Function  TreatAsAtomicUnit=on
  MATLAB Function4 : MATLAB Function  TreatAsAtomicUnit=on
  MATLAB Function5 : MATLAB Function  TreatAsAtomicUnit=on
  MATLAB Function6 : MATLAB Function  TreatAsAtomicUnit=on
  Product : Product  Multiplication=Matrix(*)
  Product1 : Product  Inputs=3  Multiplication=Matrix(*)
  Product2 : Product
  Sum : Sum  Inputs=|+-
  Sum1 : Sum  Inputs=|++
  Sum3 : Sum
  Sum4 : Sum  Inputs=--+
  T0 : Constant  Value=T0
  Transpose : Math  Operator=transpose  SaturateOnIntegerOverflow=on
  Vector Concatenate : Concatenate  Mode=Multidimensional array  ConcatenateDimension=2
  Vector Concatenate1 : Concatenate  NumInputs=3  Mode=Multidimensional array  ConcatenateDimension=2
  "[0; 0; 1]" : Constant  Value=[0; 0; 1]
  "[0; 1; 0]" : Constant  Value=[0; 1; 0]
  "[1; 0; 0]" : Constant  Value=[1; 0; 0]
  g0 : Constant  Value=g0
  m : Constant  Value=m
  pc : Constant  Value=pc
  zero : Constant  Value=0
  r : Outport
  wires:
  MATLAB Function2/1(u) -> Vector Concatenate1/3
  zero/1 -> MATLAB Function4/8(g0), MATLAB Function2/8(g0), MATLAB Function3/8(g0)
  MATLAB Function5/2(A) -> MATLAB Function6/6(A), MATLAB Function4/6(A), MATLAB Function3/6(A), MATLAB Function2/6(A)
  Sum/1 -> Product/2
  Sum1/1 -> Integrator/1
  T0/1 -> Sum4/2
  Vector Concatenate/1 -> Sum3/1
  Inertia/1 -> MATLAB Function6/5(I), MATLAB Function4/5(I), MATLAB Function3/5(I), MATLAB Function2/5(I)
  Sum4/1 -> Gain/1
  Constant/1 -> Vector Concatenate/1
  Gain/1 -> Sum1/2, r/1
  Sum3/1 -> MATLAB Function5/1(arrays)
  Constant1/1 -> MATLAB Function6/1(dq), MATLAB Function2/2(v), MATLAB Function2/1(dq), MATLAB Function3/2(v), MATLAB Function3/1(dq), MATLAB Function4/2(v), MATLAB Function4/1(dq), MATLAB Function6/2(v), MATLAB Function6/3(ddq)
  Demux3/1 -> Vector Concatenate/2
  "[1; 0; 0]"/1 -> MATLAB Function4/3(ddq)
  MATLAB Function6/1(u) -> Sum/2
  x/1 -> Demux2/1, Demux3/1
  "[0; 1; 0]"/1 -> MATLAB Function3/3(ddq)
  u_m/1 -> Sum/1
  m/1 -> MATLAB Function2/4(m), MATLAB Function3/4(m), MATLAB Function4/4(m), MATLAB Function6/4(m)
  "[0; 0; 1]"/1 -> MATLAB Function2/3(ddq)
  Constant3/1 -> Product2/2
  MATLAB Function4/1(u) -> Vector Concatenate1/1
  DHTable/1 -> Sum3/2
  MATLAB Function3/1(u) -> Vector Concatenate1/2
  Product1/1 -> Product2/1
  Vector Concatenate1/1 -> Product1/2
  Product2/1 -> Sum4/3
  g0/1 -> MATLAB Function6/8(g0)
  Demux2/2 -> Product1/3, Transpose/1
  Transpose/1 -> Product1/1, Product/1
  pc/1 -> MATLAB Function6/7(pc), MATLAB Function4/7(pc), MATLAB Function3/7(pc), MATLAB Function2/7(pc)
  Product/1 -> Sum1/1
  Integrator/1 -> Sum4/1

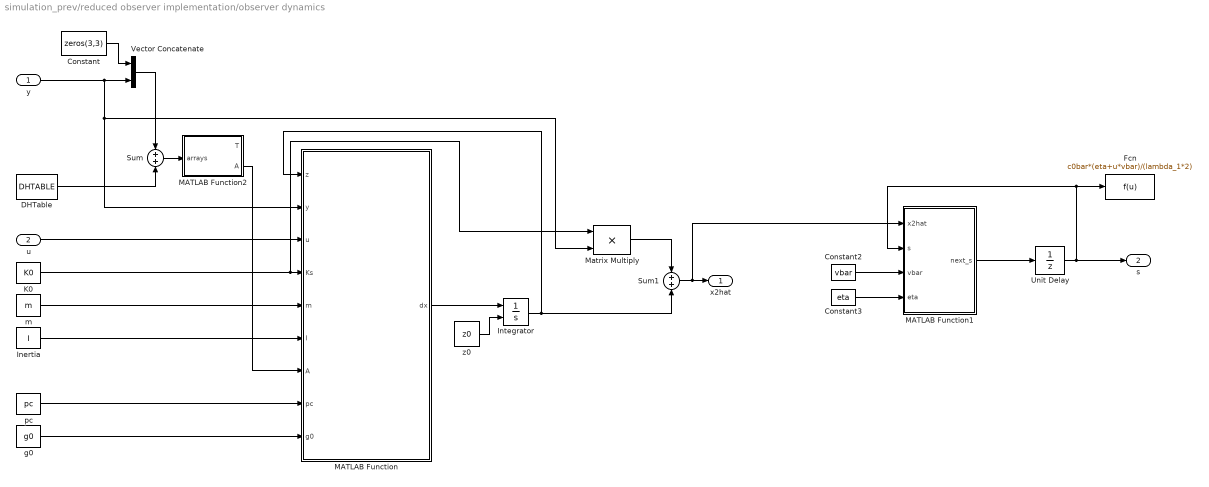
== system simulation_prev/reduced observer implementation/observer dynamics ==
  y : Inport
  u : Inport  Port=2
  Constant : Constant  Value=zeros(3,3)
  Constant2 : Constant  Value=vbar
  Constant3 : Constant  Value=eta
  DHTable : Constant  Value=DHTABLE
  Fcn : Fcn  Expr=c0bar*(eta+u*vbar)/(lambda_1*2)
  Inertia : Constant  Value=I
  Integrator : Integrator  InitialConditionSource=external  InitialCondition=[0 pi/4 pi/4 0 0 0]'
  K0 : Constant  Value=K0
  MATLAB Function : MATLAB Function  TreatAsAtomicUnit=on
  MATLAB Function1 : MATLAB Function  TreatAsAtomicUnit=on
  MATLAB Function2 : MATLAB Function  TreatAsAtomicUnit=on
  Matrix Multiply : Product
  Sum : Sum
  Sum1 : Sum
  Unit Delay : UnitDelay  InitialCondition=s0  SampleTime=-1  HasFrameUpgradeWarning=on
  Vector Concatenate : Concatenate  Mode=Multidimensional array  ConcatenateDimension=2
  g0 : Constant  Value=g0
  m : Constant  Value=m
  pc : Constant  Value=pc
  z0 : Constant  Value=z0
  x2hat : Outport
  s : Outport  Port=2
  wires:
  Sum/1 -> MATLAB Function2/1(arrays)
  u/1 -> MATLAB Function/3(u)
  pc/1 -> MATLAB Function/8(pc)
  MATLAB Function2/2(A) -> MATLAB Function/7(A)
  MATLAB Function/1(dx) -> Integrator/1
  DHTable/1 -> Sum/2
  z0/1 -> Integrator/2
  Constant/1 -> Vector Concatenate/1
  Vector Concatenate/1 -> Sum/1
  Inertia/1 -> MATLAB Function/6(I)
  g0/1 -> MATLAB Function/9(g0)
  m/1 -> MATLAB Function/5(m)
  Integrator/1 -> MATLAB Function/1(z), Sum1/2
  Sum1/1 -> MATLAB Function1/1(x2hat), x2hat/1
  Matrix Multiply/1 -> Sum1/1
  y/1 -> Vector Concatenate/2, Matrix Multiply/2, MATLAB Function/2(y)
  Constant2/1 -> MATLAB Function1/3(vbar)
  Unit Delay/1 -> s/1, MATLAB Function1/2(s), Fcn/1
  MATLAB Function1/1(next_s) -> Unit Delay/1
  Constant3/1 -> MATLAB Function1/4(eta)
  K0/1 -> Matrix Multiply/1, MATLAB Function/4(Ks)

== matlab function simulation_prev/full state implementation/energy residual/MATLAB Function5 ==
  data: arrays input; T output; A output
function [T, A] = DHMatrix(arrays)
% T = DHMatrix(arrays) takes as inputs:
%   -arrays: a n-vector of vectors composed like this: [alpha a d theta]
% and outputs:
%   -T: the product of all the matrices corresponding to each vector of arrays
% Remember that:
% cos(q1 + q2) = cos(q1)*cos(q2) - sin(q1)*sin(q2)
% sin(q1 + q2) = cos(q1)*sin(q2) + cos(q2)*sin(q1)
% making use of the simplify function these are converted automatically

    T = eye(4);
    nums = size(arrays);
    
    A = zeros(4,4,nums(1));
    
    for i = 1:nums(1)
        line = arrays(i, :);
        R = [cos(line(4)) -cos(line(1))*sin(line(4)) sin(line(1))*sin(line(4)) line(2)*cos(line(4));
             sin(line(4)) cos(line(1))*cos(line(4)) -sin(line(1))*cos(line(4)) line(2)*sin(line(4));
             0 sin(line(1)) cos(line(1)) line(3);
             0 0 0 1];
        A(:,:,i) = R;
        T = T * R;   
    end
end

== matlab function simulation_prev/full state implementation/energy residual/MATLAB Function6 ==
  data: dq input; u output; v input; ddq input; m input; I input; A input; pc input; g0 input
function u = modNE(dq,v,ddq,m,I,A,pc,g0)
% Implementation of Modified Newton-Euler algorithm

n = size(dq,1);
% check dimension consistency
if ~(size(v,1)==n && size(ddq,1)==n && size(dq,2)==1 && ...
     size(v,2)==1 && size(ddq,2)==1 && size(m,1)==n && ...
     size(I,3)==n && size(A,3)==n && size(pc,2)==n) 
    disp("Inconsistent input arguments dimension")
    u = zeros(n,1);
    return
end

% initialization
R = A(1:3,1:3,:);
p = [R(:,:,1)'*A(1:3,4,1) R(:,:,2)'*A(1:3,4,2) R(:,:,3)'*A(1:3,4,3)];
w = zeros(3,n+1);
wa = zeros(3,n+1);
dw = zeros(3,n+1);
a = zeros(3,n+1)-[[0 0 -g0]' zeros(3,n)];
ac = zeros(3,n+1);
f = zeros(3,n+1);
t = zeros(3,n+1);
u = zeros(n,1);

% forward recursion
for i = 2:n+1
   w(:,i) = R(:,:,i-1)'*(w(:,i-1)+dq(i-1)*[0 0 1]');
   wa(:,i) = R(:,:,i-1)'*(wa(:,i-1)+v(i-1)*[0 0 1]');
   dw(:,i) = R(:,:,i-1)'*(dw(:,i-1)+ddq(i-1)*[0 0 1]'+cross(dq(i-1)*wa(:,i-1),[0 0 1]'));
   a(:,i) = R(:,:,i-1)'*a(:,i-1)+cross(dw(:,i),p(:,i-1))+cross(w(:,i),cross(wa(:,i),p(:,i-1)));
   ac(:,i) = a(:,i)+cross(dw(:,i),pc(:,i-1))+cross(w(:,i),cross(wa(:,i),pc(:,i-1)));
end

w = w(:,2:n+1);
wa = wa(:,2:n+1);
dw = dw(:,2:n+1);
ac = ac(:,2:n+1);
R = cat(3,R,eye(3));

% backward recursion
for i = n:-1:1
    f(:,i) = R(:,:,i+1)*f(:,i+1)+m(i)*ac(:,i);
    t(:,i) = R(:,:,i+1)*t(:,i+1)+cross(R(:,:,i+1)*f(:,i+1),pc(:,i))-cross(f(:,i),p(:,i)+pc(:,i))+I(:,:,i)*dw(:,i)+cross(w(:,i),I(:,:,i)*wa(:,i));
    % assuming all revolute joints
    u(i) = t(:,i)'*(R(:,:,i)'*[0 0 1]');
end
end

== matlab function simulation_prev/reduced observer implementation/observer dynamics/MATLAB Function ==
  data: z input; y input; u input; Ks input; dx output; m input; I input; A input; pc input; g0 input
function dx = redobs_dynamics(z,y,u,Ks,m,I,A,pc,g0)
% return the continuous time dynamics of the reduced-order observer
% given state and input
e0 = zeros(3,1);
e1 = [1 0 0]';
e2 = [0 1 0]';
e3 = [0 0 1]';
x2hat = z + Ks*y;
%get inertia matrix M from modNE algorithm
M = [modNE(e0,e0,e1,m,I,A,pc,0) modNE(e0,e0,e2,m,I,A,pc,0) modNE(e0,e0,e3,m,I,A,pc,0)];
cg =  modNE(x2hat,x2hat,e0,m,I,A,pc,g0);
dx=inv(M)*(-cg+u)-Ks*x2hat;
end

== matlab function simulation_prev/reduced observer implementation/Controller/MATLAB Function1 ==
  data: dq input; u output; v input; ddq input; m input; I input; A input; pc input; g0 input
function u = modNE(dq,v,ddq,m,I,A,pc,g0)
% Implementation of Modified Newton-Euler algorithm

n = size(dq,1);
% check dimension consistency
if ~(size(v,1)==n && size(ddq,1)==n && size(dq,2)==1 && ...
     size(v,2)==1 && size(ddq,2)==1 && size(m,1)==n && ...
     size(I,3)==n && size(A,3)==n && size(pc,2)==n) 
    disp("Inconsistent input arguments dimension")
    u = zeros(n,1);
    return
end

% initialization
R = A(1:3,1:3,:);
p = [R(:,:,1)'*A(1:3,4,1) R(:,:,2)'*A(1:3,4,2) R(:,:,3)'*A(1:3,4,3)];
w = zeros(3,n+1);
wa = zeros(3,n+1);
dw = zeros(3,n+1);
a = zeros(3,n+1)-[[0 0 -g0]' zeros(3,n)];
ac = zeros(3,n+1);
f = zeros(3,n+1);
t = zeros(3,n+1);
u = zeros(n,1);

% forward recursion
for i = 2:n+1
   w(:,i) = R(:,:,i-1)'*(w(:,i-1)+dq(i-1)*[0 0 1]');
   wa(:,i) = R(:,:,i-1)'*(wa(:,i-1)+v(i-1)*[0 0 1]');
   dw(:,i) = R(:,:,i-1)'*(dw(:,i-1)+ddq(i-1)*[0 0 1]'+cross(dq(i-1)*wa(:,i-1),[0 0 1]'));
   a(:,i) = R(:,:,i-1)'*a(:,i-1)+cross(dw(:,i),p(:,i-1))+cross(w(:,i),cross(wa(:,i),p(:,i-1)));
   ac(:,i) = a(:,i)+cross(dw(:,i),pc(:,i-1))+cross(w(:,i),cross(wa(:,i),pc(:,i-1)));
end

w = w(:,2:n+1);
wa = wa(:,2:n+1);
dw = dw(:,2:n+1);
ac = ac(:,2:n+1);
R = cat(3,R,eye(3));

% backward recursion
for i = n:-1:1
    f(:,i) = R(:,:,i+1)*f(:,i+1)+m(i)*ac(:,i);
    t(:,i) = R(:,:,i+1)*t(:,i+1)+cross(R(:,:,i+1)*f(:,i+1),pc(:,i))-cross(f(:,i),p(:,i)+pc(:,i))+I(:,:,i)*dw(:,i)+cross(w(:,i),I(:,:,i)*wa(:,i));
    % assuming all revolute joints
    u(i) = t(:,i)'*(R(:,:,i)'*[0 0 1]');
end
end

== matlab function simulation_prev/reduced observer implementation/observer dynamics/MATLAB Function2 ==
  data: arrays input; T output; A output
function [T, A] = DHMatrix(arrays)
% T = DHMatrix(arrays) takes as inputs:
%   -arrays: a n-vector of vectors composed like this: [alpha a d theta]
% and outputs:
%   -T: the product of all the matrices corresponding to each vector of arrays
% Remember that:
% cos(q1 + q2) = cos(q1)*cos(q2) - sin(q1)*sin(q2)
% sin(q1 + q2) = cos(q1)*sin(q2) + cos(q2)*sin(q1)
% making use of the simplify function these are converted automatically

    T = eye(4);
    nums = size(arrays);
    
    A = zeros(4,4,nums(1));
    
    for i = 1:nums(1)
        line = arrays(i, :);
        R = [cos(line(4)) -cos(line(1))*sin(line(4)) sin(line(1))*sin(line(4)) line(2)*cos(line(4));
             sin(line(4)) cos(line(1))*cos(line(4)) -sin(line(1))*cos(line(4)) line(2)*sin(line(4));
             0 sin(line(1)) cos(line(1)) line(3);
             0 0 0 1];
        A(:,:,i) = R;
        T = T * R;   
    end
end

== matlab function simulation_prev/reduced observer implementation/Controller/MATLAB Function3 ==
  data: arrays input; T output; A output
function [T, A] = DHMatrix(arrays)
% T = DHMatrix(arrays) takes as inputs:
%   -arrays: a n-vector of vectors composed like this: [alpha a d theta]
% and outputs:
%   -T: the product of all the matrices corresponding to each vector of arrays
% Remember that:
% cos(q1 + q2) = cos(q1)*cos(q2) - sin(q1)*sin(q2)
% sin(q1 + q2) = cos(q1)*sin(q2) + cos(q2)*sin(q1)
% making use of the simplify function these are converted automatically

    T = eye(4);
    nums = size(arrays);
    
    A = zeros(4,4,nums(1));
    
    for i = 1:nums(1)
        line = arrays(i, :);
        R = [cos(line(4)) -cos(line(1))*sin(line(4)) sin(line(1))*sin(line(4)) line(2)*cos(line(4));
             sin(line(4)) cos(line(1))*cos(line(4)) -sin(line(1))*cos(line(4)) line(2)*sin(line(4));
             0 sin(line(1)) cos(line(1)) line(3);
             0 0 0 1];
        A(:,:,i) = R;
        T = T * R;   
    end
end

== matlab function simulation_prev/full state implementation/Controller/MATLAB Function1 ==
  data: dq input; u output; v input; ddq input; m input; I input; A input; pc input; g0 input
function u = modNE(dq,v,ddq,m,I,A,pc,g0)
% Implementation of Modified Newton-Euler algorithm

n = size(dq,1);
% check dimension consistency
if ~(size(v,1)==n && size(ddq,1)==n && size(dq,2)==1 && ...
     size(v,2)==1 && size(ddq,2)==1 && size(m,1)==n && ...
     size(I,3)==n && size(A,3)==n && size(pc,2)==n) 
    disp("Inconsistent input arguments dimension")
    u = zeros(n,1);
    return
end

% initialization
R = A(1:3,1:3,:);
p = [R(:,:,1)'*A(1:3,4,1) R(:,:,2)'*A(1:3,4,2) R(:,:,3)'*A(1:3,4,3)];
w = zeros(3,n+1);
wa = zeros(3,n+1);
dw = zeros(3,n+1);
a = zeros(3,n+1)-[[0 0 -g0]' zeros(3,n)];
ac = zeros(3,n+1);
f = zeros(3,n+1);
t = zeros(3,n+1);
u = zeros(n,1);

% forward recursion
for i = 2:n+1
   w(:,i) = R(:,:,i-1)'*(w(:,i-1)+dq(i-1)*[0 0 1]');
   wa(:,i) = R(:,:,i-1)'*(wa(:,i-1)+v(i-1)*[0 0 1]');
   dw(:,i) = R(:,:,i-1)'*(dw(:,i-1)+ddq(i-1)*[0 0 1]'+cross(dq(i-1)*wa(:,i-1),[0 0 1]'));
   a(:,i) = R(:,:,i-1)'*a(:,i-1)+cross(dw(:,i),p(:,i-1))+cross(w(:,i),cross(wa(:,i),p(:,i-1)));
   ac(:,i) = a(:,i)+cross(dw(:,i),pc(:,i-1))+cross(w(:,i),cross(wa(:,i),pc(:,i-1)));
end

w = w(:,2:n+1);
wa = wa(:,2:n+1);
dw = dw(:,2:n+1);
ac = ac(:,2:n+1);
R = cat(3,R,eye(3));

% backward recursion
for i = n:-1:1
    f(:,i) = R(:,:,i+1)*f(:,i+1)+m(i)*ac(:,i);
    t(:,i) = R(:,:,i+1)*t(:,i+1)+cross(R(:,:,i+1)*f(:,i+1),pc(:,i))-cross(f(:,i),p(:,i)+pc(:,i))+I(:,:,i)*dw(:,i)+cross(w(:,i),I(:,:,i)*wa(:,i));
    % assuming all revolute joints
    u(i) = t(:,i)'*(R(:,:,i)'*[0 0 1]');
end
end

== matlab function simulation_prev/reduced observer implementation/Robot dynamics/MATLAB Function ==
  data: x input; u input; dx output; m input; I input; A input; pc input; g0 input
function dx = ct_dynamics(x,u,m,I,A,pc,g0)
% return the continuous time dynamics given state and input
e0 = zeros(3,1);
e1 = [1 0 0]';
e2 = [0 1 0]';
e3 = [0 0 1]';
x2 = x(4:6);
%get inertia matrix M from modNE algorithm
M = [modNE(e0,e0,e1,m,I,A,pc,0) modNE(e0,e0,e2,m,I,A,pc,0) modNE(e0,e0,e3,m,I,A,pc,0)];
iM = inv(M);
cg =  modNE(x2,x2,e0,m,I,A,pc,g0);
dx=[x2;
    iM*(-cg+u)];
end

== matlab function simulation_prev/reduced observer implementation/Robot dynamics/MATLAB Function2 ==
  data: arrays input; T output; A output
function [T, A] = DHMatrix(arrays)
% T = DHMatrix(arrays) takes as inputs:
%   -arrays: a n-vector of vectors composed like this: [alpha a d theta]
% and outputs:
%   -T: the product of all the matrices corresponding to each vector of arrays
% Remember that:
% cos(q1 + q2) = cos(q1)*cos(q2) - sin(q1)*sin(q2)
% sin(q1 + q2) = cos(q1)*sin(q2) + cos(q2)*sin(q1)
% making use of the simplify function these are converted automatically

    T = eye(4);
    nums = size(arrays);
    
    A = zeros(4,4,nums(1));
    
    for i = 1:nums(1)
        line = arrays(i, :);
        R = [cos(line(4)) -cos(line(1))*sin(line(4)) sin(line(1))*sin(line(4)) line(2)*cos(line(4));
             sin(line(4)) cos(line(1))*cos(line(4)) -sin(line(1))*cos(line(4)) line(2)*sin(line(4));
             0 sin(line(1)) cos(line(1)) line(3);
             0 0 0 1];
        A(:,:,i) = R;
        T = T * R;   
    end
end

== matlab function simulation_prev/reduced observer implementation/energy residual/MATLAB Function2 ==
  data: dq input; u output; v input; ddq input; m input; I input; A input; pc input; g0 input
function u = modNE(dq,v,ddq,m,I,A,pc,g0)
% Implementation of Modified Newton-Euler algorithm

n = size(dq,1);
% check dimension consistency
if ~(size(v,1)==n && size(ddq,1)==n && size(dq,2)==1 && ...
     size(v,2)==1 && size(ddq,2)==1 && size(m,1)==n && ...
     size(I,3)==n && size(A,3)==n && size(pc,2)==n) 
    disp("Inconsistent input arguments dimension")
    u = zeros(n,1);
    return
end

% initialization
R = A(1:3,1:3,:);
p = [R(:,:,1)'*A(1:3,4,1) R(:,:,2)'*A(1:3,4,2) R(:,:,3)'*A(1:3,4,3)];
w = zeros(3,n+1);
wa = zeros(3,n+1);
dw = zeros(3,n+1);
a = zeros(3,n+1)-[[0 0 -g0]' zeros(3,n)];
ac = zeros(3,n+1);
f = zeros(3,n+1);
t = zeros(3,n+1);
u = zeros(n,1);

% forward recursion
for i = 2:n+1
   w(:,i) = R(:,:,i-1)'*(w(:,i-1)+dq(i-1)*[0 0 1]');
   wa(:,i) = R(:,:,i-1)'*(wa(:,i-1)+v(i-1)*[0 0 1]');
   dw(:,i) = R(:,:,i-1)'*(dw(:,i-1)+ddq(i-1)*[0 0 1]'+cross(dq(i-1)*wa(:,i-1),[0 0 1]'));
   a(:,i) = R(:,:,i-1)'*a(:,i-1)+cross(dw(:,i),p(:,i-1))+cross(w(:,i),cross(wa(:,i),p(:,i-1)));
   ac(:,i) = a(:,i)+cross(dw(:,i),pc(:,i-1))+cross(w(:,i),cross(wa(:,i),pc(:,i-1)));
end

w = w(:,2:n+1);
wa = wa(:,2:n+1);
dw = dw(:,2:n+1);
ac = ac(:,2:n+1);
R = cat(3,R,eye(3));

% backward recursion
for i = n:-1:1
    f(:,i) = R(:,:,i+1)*f(:,i+1)+m(i)*ac(:,i);
    t(:,i) = R(:,:,i+1)*t(:,i+1)+cross(R(:,:,i+1)*f(:,i+1),pc(:,i))-cross(f(:,i),p(:,i)+pc(:,i))+I(:,:,i)*dw(:,i)+cross(w(:,i),I(:,:,i)*wa(:,i));
    % assuming all revolute joints
    u(i) = t(:,i)'*(R(:,:,i)'*[0 0 1]');
end
end

== matlab function simulation_prev/reduced observer implementation/energy residual/MATLAB Function3 ==
  data: dq input; u output; v input; ddq input; m input; I input; A input; pc input; g0 input
function u = modNE(dq,v,ddq,m,I,A,pc,g0)
% Implementation of Modified Newton-Euler algorithm

n = size(dq,1);
% check dimension consistency
if ~(size(v,1)==n && size(ddq,1)==n && size(dq,2)==1 && ...
     size(v,2)==1 && size(ddq,2)==1 && size(m,1)==n && ...
     size(I,3)==n && size(A,3)==n && size(pc,2)==n) 
    disp("Inconsistent input arguments dimension")
    u = zeros(n,1);
    return
end

% initialization
R = A(1:3,1:3,:);
p = [R(:,:,1)'*A(1:3,4,1) R(:,:,2)'*A(1:3,4,2) R(:,:,3)'*A(1:3,4,3)];
w = zeros(3,n+1);
wa = zeros(3,n+1);
dw = zeros(3,n+1);
a = zeros(3,n+1)-[[0 0 -g0]' zeros(3,n)];
ac = zeros(3,n+1);
f = zeros(3,n+1);
t = zeros(3,n+1);
u = zeros(n,1);

% forward recursion
for i = 2:n+1
   w(:,i) = R(:,:,i-1)'*(w(:,i-1)+dq(i-1)*[0 0 1]');
   wa(:,i) = R(:,:,i-1)'*(wa(:,i-1)+v(i-1)*[0 0 1]');
   dw(:,i) = R(:,:,i-1)'*(dw(:,i-1)+ddq(i-1)*[0 0 1]'+cross(dq(i-1)*wa(:,i-1),[0 0 1]'));
   a(:,i) = R(:,:,i-1)'*a(:,i-1)+cross(dw(:,i),p(:,i-1))+cross(w(:,i),cross(wa(:,i),p(:,i-1)));
   ac(:,i) = a(:,i)+cross(dw(:,i),pc(:,i-1))+cross(w(:,i),cross(wa(:,i),pc(:,i-1)));
end

w = w(:,2:n+1);
wa = wa(:,2:n+1);
dw = dw(:,2:n+1);
ac = ac(:,2:n+1);
R = cat(3,R,eye(3));

% backward recursion
for i = n:-1:1
    f(:,i) = R(:,:,i+1)*f(:,i+1)+m(i)*ac(:,i);
    t(:,i) = R(:,:,i+1)*t(:,i+1)+cross(R(:,:,i+1)*f(:,i+1),pc(:,i))-cross(f(:,i),p(:,i)+pc(:,i))+I(:,:,i)*dw(:,i)+cross(w(:,i),I(:,:,i)*wa(:,i));
    % assuming all revolute joints
    u(i) = t(:,i)'*(R(:,:,i)'*[0 0 1]');
end
end

== matlab function simulation_prev/reduced observer implementation/energy residual/MATLAB Function4 ==
  data: dq input; u output; v input; ddq input; m input; I input; A input; pc input; g0 input
function u = modNE(dq,v,ddq,m,I,A,pc,g0)
% Implementation of Modified Newton-Euler algorithm

n = size(dq,1);
% check dimension consistency
if ~(size(v,1)==n && size(ddq,1)==n && size(dq,2)==1 && ...
     size(v,2)==1 && size(ddq,2)==1 && size(m,1)==n && ...
     size(I,3)==n && size(A,3)==n && size(pc,2)==n) 
    disp("Inconsistent input arguments dimension")
    u = zeros(n,1);
    return
end

% initialization
R = A(1:3,1:3,:);
p = [R(:,:,1)'*A(1:3,4,1) R(:,:,2)'*A(1:3,4,2) R(:,:,3)'*A(1:3,4,3)];
w = zeros(3,n+1);
wa = zeros(3,n+1);
dw = zeros(3,n+1);
a = zeros(3,n+1)-[[0 0 -g0]' zeros(3,n)];
ac = zeros(3,n+1);
f = zeros(3,n+1);
t = zeros(3,n+1);
u = zeros(n,1);

% forward recursion
for i = 2:n+1
   w(:,i) = R(:,:,i-1)'*(w(:,i-1)+dq(i-1)*[0 0 1]');
   wa(:,i) = R(:,:,i-1)'*(wa(:,i-1)+v(i-1)*[0 0 1]');
   dw(:,i) = R(:,:,i-1)'*(dw(:,i-1)+ddq(i-1)*[0 0 1]'+cross(dq(i-1)*wa(:,i-1),[0 0 1]'));
   a(:,i) = R(:,:,i-1)'*a(:,i-1)+cross(dw(:,i),p(:,i-1))+cross(w(:,i),cross(wa(:,i),p(:,i-1)));
   ac(:,i) = a(:,i)+cross(dw(:,i),pc(:,i-1))+cross(w(:,i),cross(wa(:,i),pc(:,i-1)));
end

w = w(:,2:n+1);
wa = wa(:,2:n+1);
dw = dw(:,2:n+1);
ac = ac(:,2:n+1);
R = cat(3,R,eye(3));

% backward recursion
for i = n:-1:1
    f(:,i) = R(:,:,i+1)*f(:,i+1)+m(i)*ac(:,i);
    t(:,i) = R(:,:,i+1)*t(:,i+1)+cross(R(:,:,i+1)*f(:,i+1),pc(:,i))-cross(f(:,i),p(:,i)+pc(:,i))+I(:,:,i)*dw(:,i)+cross(w(:,i),I(:,:,i)*wa(:,i));
    % assuming all revolute joints
    u(i) = t(:,i)'*(R(:,:,i)'*[0 0 1]');
end
end
